simulink model "Wrapper_seat_heating_control"  (R2022b)
settings: Solver=FixedStepDiscrete  StartTime=0.0  StopTime=10.0  FixedStep=0.01  RelTol=1e-3
undefined symbols (not defined in the file or in its folder): ep_dummy_code_func, HeatingActivate_SetHeatingCoil, temp
settings Model: Tag=EP_AUTOSAR_SWC_WRAPPER_COMPLETE  Creator=developer  LastModifiedBy=developer
settings SolverCC: AlgebraicLoopSolver=TrustRegion
settings DataIOCC: SaveFormat=StructureWithTime
settings OptimizationCC: DefaultParameterBehavior=Inlined  EnhancedBackFolding=on  PassReuseOutputArgsAs=Individual arguments  ZeroExternalMemoryAtStartup=off  ZeroInternalMemoryAtStartup=off  OptimizeBlockOrder=speed  DifferentSizesBufferReuse=on  OptimizationCustomize=off  EfficientTunableParamExpr=on
settings DebuggingCC: ParameterTunabilityLossMsg=error  UnconnectedInputMsg=warning  UnconnectedOutputMsg=warning  UnconnectedLineMsg=warning  SFMachineParentedDataDiag=warning  ArithmeticOperatorsInVariantConditions=warning
settings ModelReferenceCC: ModelReferenceNumInstancesAllowed=Single
settings SFSimCC: MATLABDynamicMemAlloc=off  CustomCodeUndefinedFunction=UseInterfaceOnly
settings RTWCC: Description=Embedded Coder  SystemTargetFile=ert.tlc  GenCodeOnly=on  TemplateMakefile=ert_default_tmf  GenerateReport=on  IncludeHyperlinkInReport=on  LaunchReport=on  GenerateTraceInfo=on  GenerateTraceReport=on  GenerateTraceReportSl=on  GenerateTraceReportSf=on  GenerateTraceReportEml=on
settings RTWCC: CustomSourceCode=|
  | /* BTC-EP -- stub implementation for dummy function */
  | void dummy_caller_rte_funcs() {}
settings RTWCC: CustomHeaderCode=|
  | /* BTC-EP -- include the AUTOSAR model RTE header for the init function */
  | #include "Rte_SeatHeatControl.h"
settings RTWCC: CustomInitializer=|
  | /* BTC-EP -- call the AUTOSAR model init function */
  | SeatHeatControl_Init();
settings CodeAppCC: ForceParamTrailComments=on  IgnoreCustomStorageClasses=off  MaxIdLength=256  OperatorAnnotations=on  SimulinkDataObjDesc=on  SFDataObjDesc=on  CustomSymbolStrGlobalVar=w_$R$N$M  CustomSymbolStrType=w_$N$R$M_T  InsertBlockDesc=on
settings ERTTargetCC: TargetLangStandard=C99 (ISO)  GenerateSampleERTMain=on  InlinedParameterPlacement=NonHierarchical  ERTCustomFileTemplate=example_file_process.tlc

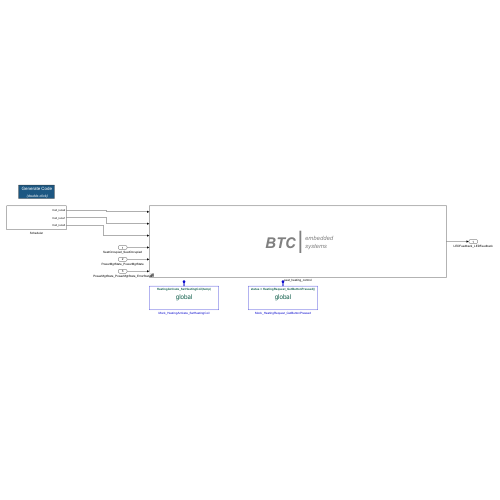
[thumbnail: Simulink's stored preview of the top-level diagram]
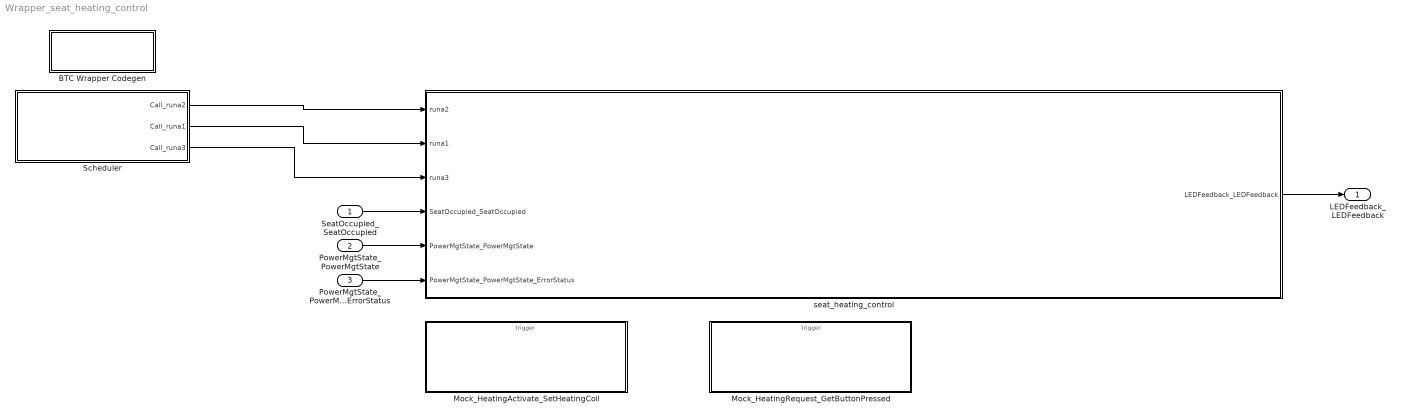
== system Wrapper_seat_heating_control ==
  SeatOccupied_SeatOccupied : Inport  OutDataTypeStr=IDT_SeatStatus  PortDimensions=1
  PowerMgtState_PowerMgtState : Inport  Port=2  OutDataTypeStr=Enum: IDT_PowerState  PortDimensions=1
  PowerMgtState_PowerMgtState_ErrorStatus : Inport  Port=3  OutDataTypeStr=uint8  PortDimensions=1
  BTC Wrapper Codegen : Subsystem  mask(BTC Wrapper Codegen Block){}
      settings: OpenFcn=ep_core_feval('ep_ec_model_callbacks', gcbh);
      mask DialogControl DescGroupVar Prompt: BTC Codegen
      mask DialogControl DescTextVar Prompt: This is the BTC Embedded Systems Wrapper Codegen block.By double-clicking this block, code will be generated for the referenced model and the wrapper.
      mask Display: disp('\color{white}\fontsize{15} Generate Code\newline \color{white}\it\fontsize{12}     (double-click)', 'texmode', 'on');
  Mock_HeatingActivate_SetHeatingCoil : Subsystem  TreatAsAtomicUnit=on
  Mock_HeatingRequest_GetButtonPressed : Subsystem  TreatAsAtomicUnit=on
  Scheduler : Subsystem
  seat_heating_control : Subsystem  Variant=on  VariantControlMode=label  LabelModeActiveChoice=orig  PropagateVariantConditions=on
      mask DialogControl DescGroupVar Prompt: BTC Embedded Systems SUT block
      mask DialogControl DescTextVar Prompt: This is the BTC Embedded Systems SUT block, referencing the original AUTOSAR model.
      mask Display: disp('\color{gray}\it\fontsize{20}                          embedded\newline                          systems', 'texmode', 'on');disp('{{\color{gray}\bf\fontsize{50}\it   BTC}  \fontsize{80}|      \color{black}\fontsize{20}\newline }', 'texmode','on');
  LEDFeedback_LEDFeedback : Outport  OutDataTypeStr=boolean  PortDimensions=3
  wires:
  SeatOccupied_SeatOccupied/1 -> seat_heating_control/4(SeatOccupied_SeatOccupied)
  PowerMgtState_PowerMgtState/1 -> seat_heating_control/5(PowerMgtState_PowerMgtState)
  PowerMgtState_PowerMgtState_ErrorStatus/1 -> seat_heating_control/6(PowerMgtState_PowerMgtState_ErrorStatus)
  seat_heating_control/1(LEDFeedback_LEDFeedback) -> LEDFeedback_LEDFeedback/1
  Scheduler/2(Call_runa1) -> seat_heating_control/2(runa1)
  Scheduler/1(Call_runa2) -> seat_heating_control/1(runa2)
  Scheduler/3(Call_runa3) -> seat_heating_control/3(runa3)

== system Wrapper_seat_heating_control/BTC Wrapper Codegen ==

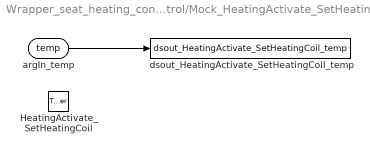
== system Wrapper_seat_heating_control/Mock_HeatingActivate_SetHeatingCoil ==
  HeatingActivate_SetHeatingCoil : TriggerPort  TriggerType=function-call  IsSimulinkFunction=on  FunctionName=HeatingActivate_SetHeatingCoil  VariantControl=(inherit)
  dsout_HeatingActivate_SetHeatingCoil_temp : DataStoreWrite  DataStoreName=dsout_HeatingActivate_SetHeatingCoil_temp  IndexOptions=Index vector (dialog)  Indices=1  OutputSizes=1
  argIn_temp : ArgIn  OutDataTypeStr=IDT_Temperature  PortDimensions="[1  1]"  ArgumentName=temp
  wires:
  argIn_temp/1 -> dsout_HeatingActivate_SetHeatingCoil_temp/1

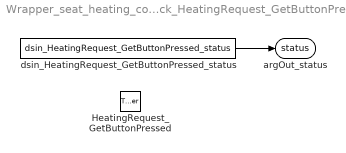
== system Wrapper_seat_heating_control/Mock_HeatingRequest_GetButtonPressed ==
  HeatingRequest_GetButtonPressed : TriggerPort  TriggerType=function-call  IsSimulinkFunction=on  FunctionName=HeatingRequest_GetButtonPressed  VariantControl=(inherit)
  dsin_HeatingRequest_GetButtonPressed_status : DataStoreRead  DataStoreName=dsin_HeatingRequest_GetButtonPressed_status  IndexOptions=Index vector (dialog)  Indices=1  OutputSizes=1
  argOut_status : ArgOut  OutDataTypeStr=IDT_ButtonStatus  PortDimensions="[1  1]"  ArgumentName=status
  wires:
  dsin_HeatingRequest_GetButtonPressed_status/1 -> argOut_status/1

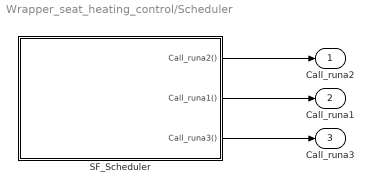
== system Wrapper_seat_heating_control/Scheduler ==
  SF_Scheduler : Stateflow chart  TreatAsAtomicUnit=on
  Call_runa2 : Outport
  Call_runa1 : Outport  Port=2
  Call_runa3 : Outport  Port=3
  wires:
  SF_Scheduler/1(Call_runa2()) -> Call_runa2/1
  SF_Scheduler/2(Call_runa1()) -> Call_runa1/1
  SF_Scheduler/3(Call_runa3()) -> Call_runa3/1

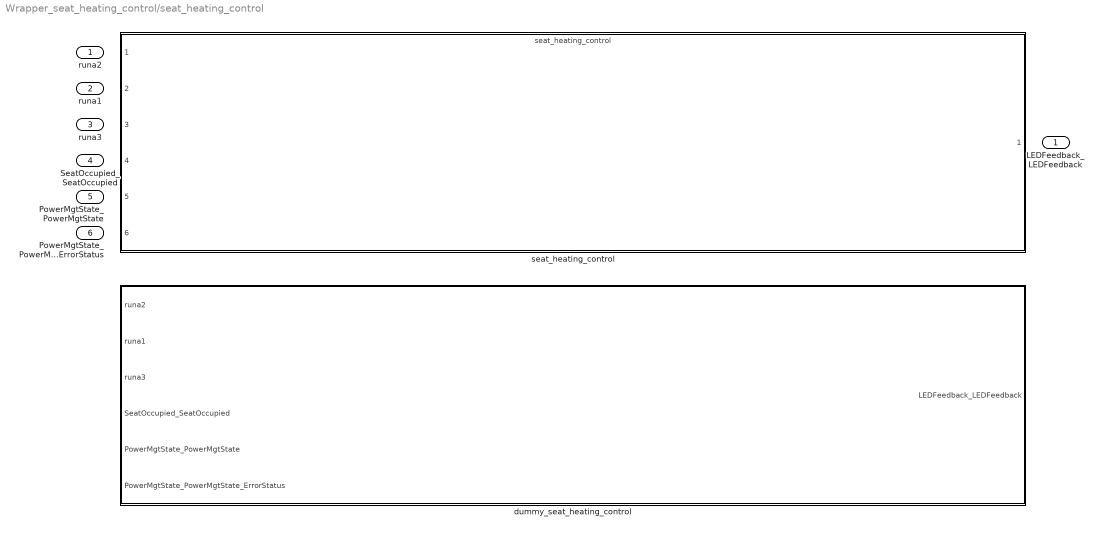
== system Wrapper_seat_heating_control/seat_heating_control ==
  runa2 : Inport
  runa1 : Inport  Port=2
  runa3 : Inport  Port=3
  SeatOccupied_SeatOccupied : Inport  Port=4
  PowerMgtState_PowerMgtState : Inport  Port=5
  PowerMgtState_PowerMgtState_ErrorStatus : Inport  Port=6
  dummy_seat_heating_control : Subsystem  VariantControl=dummy
  seat_heating_control : ModelReference  Tag=BTC AUTOSAR Main Model Reference Block  ModelNameDialog=seat_heating_control  SimulationMode=Normal  ScheduleRates=on  VariantControl=orig  ModelReferenceVersion=1.0
  LEDFeedback_LEDFeedback : Outport

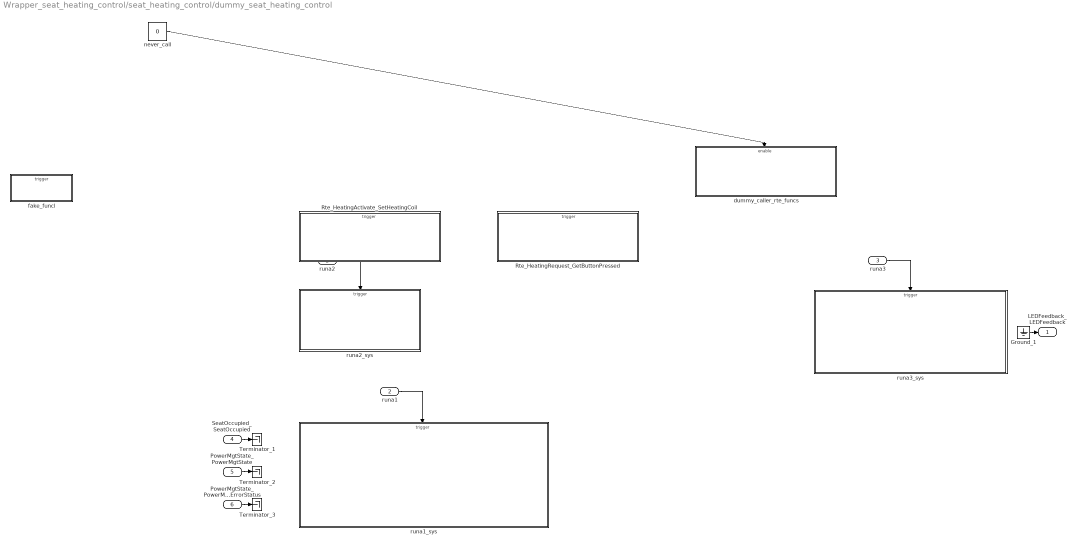
== system Wrapper_seat_heating_control/seat_heating_control/dummy_seat_heating_control ==
  runa2 : Inport  OutputFunctionCall=on
  runa1 : Inport  Port=2  OutputFunctionCall=on
  runa3 : Inport  Port=3  OutputFunctionCall=on
  SeatOccupied_SeatOccupied : Inport  Port=4  OutDataTypeStr=IDT_SeatStatus  PortDimensions=1
  PowerMgtState_PowerMgtState : Inport  Port=5  OutDataTypeStr=Enum: IDT_PowerState  PortDimensions=1
  PowerMgtState_PowerMgtState_ErrorStatus : Inport  Port=6  OutDataTypeStr=uint8  PortDimensions=1
  Ground_1 : Ground
  Rte_HeatingActivate_SetHeatingCoil : Subsystem  TreatAsAtomicUnit=on
  Rte_HeatingRequest_GetButtonPressed : Subsystem  TreatAsAtomicUnit=on
  Terminator_1 : Terminator
  Terminator_2 : Terminator
  Terminator_3 : Terminator
  dummy_caller_rte_funcs : Subsystem  TreatAsAtomicUnit=on  RTWFcnName=dummy_caller_rte_funcs  RTWFileName=ep_dummy_code
      settings: RTWSystemCode=Nonreusable function  RTWFcnNameOpts=User specified  RTWFileNameOpts=User specified
  fake_funcl : Subsystem  TreatAsAtomicUnit=on
  never_call : Constant  Value=0
  runa1_sys : Subsystem  RTWFcnName=runa1  RTWFileName=ep_dummy_code
      settings: RTWSystemCode=Nonreusable function  RTWFcnNameOpts=User specified  RTWFileNameOpts=User specified
  runa2_sys : Subsystem  RTWFcnName=runa2  RTWFileName=ep_dummy_code
      settings: RTWSystemCode=Nonreusable function  RTWFcnNameOpts=User specified  RTWFileNameOpts=User specified
  runa3_sys : Subsystem  RTWFcnName=runa3  RTWFileName=ep_dummy_code
      settings: RTWSystemCode=Nonreusable function  RTWFcnNameOpts=User specified  RTWFileNameOpts=User specified
  LEDFeedback_LEDFeedback : Outport  OutDataTypeStr=boolean  PortDimensions=3
  wires:
  runa2/1 -> runa2_sys/Trigger
  runa1/1 -> runa1_sys/Trigger
  runa3/1 -> runa3_sys/Trigger
  never_call/1 -> dummy_caller_rte_funcs/Enable
  SeatOccupied_SeatOccupied/1 -> Terminator_1/1
  PowerMgtState_PowerMgtState/1 -> Terminator_2/1
  PowerMgtState_PowerMgtState_ErrorStatus/1 -> Terminator_3/1
  Ground_1/1 -> LEDFeedback_LEDFeedback/1

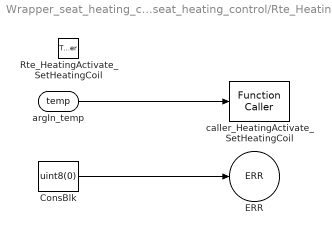
== system Wrapper_seat_heating_control/seat_heating_control/dummy_seat_heating_control/Rte_HeatingActivate_SetHeatingCoil ==
  Rte_HeatingActivate_SetHeatingCoil : TriggerPort  TriggerType=function-call  IsSimulinkFunction=on  FunctionName=Rte_HeatingActivate_SetHeatingCoil  VariantControl=(inherit)
  ConsBlk : Constant  Value=uint8(0)
  caller_HeatingActivate_SetHeatingCoil : FunctionCaller  FunctionPrototype=HeatingActivate_SetHeatingCoil(temp)  InputArgumentSpecifications=uint8(0)  OutputArgumentSpecifications=<Enter example>
  argIn_temp : ArgIn  OutDataTypeStr=IDT_Temperature  PortDimensions="[1  1]"  ArgumentName=temp
  ERR : ArgOut  OutDataTypeStr=uint8  ArgumentName=ERR
  wires:
  ConsBlk/1 -> ERR/1
  argIn_temp/1 -> caller_HeatingActivate_SetHeatingCoil/1

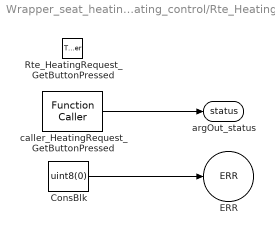
== system Wrapper_seat_heating_control/seat_heating_control/dummy_seat_heating_control/Rte_HeatingRequest_GetButtonPressed ==
  Rte_HeatingRequest_GetButtonPressed : TriggerPort  TriggerType=function-call  IsSimulinkFunction=on  FunctionName=Rte_HeatingRequest_GetButtonPressed  VariantControl=(inherit)
  ConsBlk : Constant  Value=uint8(0)
  caller_HeatingRequest_GetButtonPressed : FunctionCaller  FunctionPrototype=status = HeatingRequest_GetButtonPressed()  InputArgumentSpecifications=<Enter example>  OutputArgumentSpecifications=false
  argOut_status : ArgOut  OutDataTypeStr=IDT_ButtonStatus  PortDimensions="[1  1]"  ArgumentName=status
  ERR : ArgOut  Port=2  OutDataTypeStr=uint8  ArgumentName=ERR
  wires:
  caller_HeatingRequest_GetButtonPressed/1 -> argOut_status/1
  ConsBlk/1 -> ERR/1

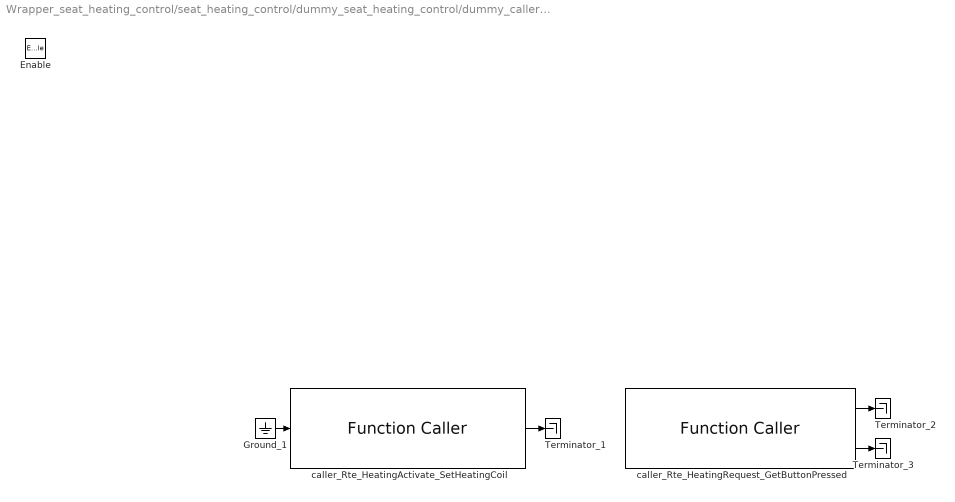
== system Wrapper_seat_heating_control/seat_heating_control/dummy_seat_heating_control/dummy_caller_rte_funcs ==
  Enable : EnablePort
  Ground_1 : Ground
  Terminator_1 : Terminator
  Terminator_2 : Terminator
  Terminator_3 : Terminator
  caller_Rte_HeatingActivate_SetHeatingCoil : FunctionCaller  FunctionPrototype=ERR = Rte_HeatingActivate_SetHeatingCoil(temp)  InputArgumentSpecifications=uint8(0)  OutputArgumentSpecifications=uint8(0)
  caller_Rte_HeatingRequest_GetButtonPressed : FunctionCaller  FunctionPrototype=[status,ERR] = Rte_HeatingRequest_GetButtonPressed()  InputArgumentSpecifications=<Enter example>  OutputArgumentSpecifications=false, uint8(0)  SampleTime=0.01
  wires:
  Ground_1/1 -> caller_Rte_HeatingActivate_SetHeatingCoil/1
  caller_Rte_HeatingActivate_SetHeatingCoil/1 -> Terminator_1/1
  caller_Rte_HeatingRequest_GetButtonPressed/1 -> Terminator_2/1
  caller_Rte_HeatingRequest_GetButtonPressed/2 -> Terminator_3/1

== system Wrapper_seat_heating_control/seat_heating_control/dummy_seat_heating_control/fake_funcl ==
  ep_dummy_code_func : TriggerPort  TriggerType=function-call  IsSimulinkFunction=on  FunctionName=ep_dummy_code_func  VariantControl=(inherit)

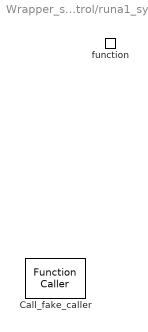
== system Wrapper_seat_heating_control/seat_heating_control/dummy_seat_heating_control/runa1_sys ==
  function : TriggerPort  TriggerType=function-call  VariantControl=(inherit)  SampleTimeType=periodic  SampleTime=-1
  Call_fake_caller : FunctionCaller  FunctionPrototype=ep_dummy_code_func()  InputArgumentSpecifications=<Enter example>  OutputArgumentSpecifications=<Enter example>

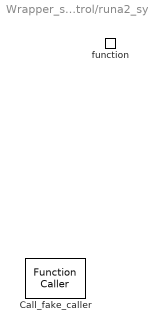
== system Wrapper_seat_heating_control/seat_heating_control/dummy_seat_heating_control/runa2_sys ==
  function : TriggerPort  TriggerType=function-call  VariantControl=(inherit)  SampleTimeType=periodic  SampleTime=-1
  Call_fake_caller : FunctionCaller  FunctionPrototype=ep_dummy_code_func()  InputArgumentSpecifications=<Enter example>  OutputArgumentSpecifications=<Enter example>

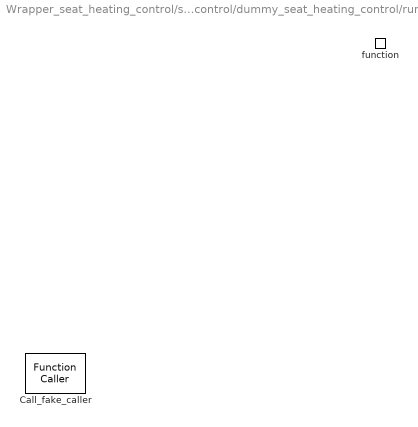
== system Wrapper_seat_heating_control/seat_heating_control/dummy_seat_heating_control/runa3_sys ==
  function : TriggerPort  TriggerType=function-call  VariantControl=(inherit)  SampleTimeType=periodic  SampleTime=-1
  Call_fake_caller : FunctionCaller  FunctionPrototype=ep_dummy_code_func()  InputArgumentSpecifications=<Enter example>  OutputArgumentSpecifications=<Enter example>

== stateflow chart Wrapper_seat_heating_control/Scheduler/SF_Scheduler ==
  state Schedule
    en:
    send(Call_runa2);
    send(Call_runa1);
    send(Call_runa3);
    du:
    on every(1, tick):send(Call_runa2);
    on every(1, tick):send(Call_runa1);
    on every(1, tick):send(Call_runa3);
  (default) -> Schedule : /*Update the Order/Rate/Asynchronous calls of the runnables*/
  events: Call_runa2 output FUNCTION_CALL_EVENT; Call_runa1 output FUNCTION_CALL_EVENT; Call_runa3 output FUNCTION_CALL_EVENT
